simulink model "Clase_parcial_2_control_2"  (R2016a)
settings: Solver=VariableStepAuto  StartTime=0.0  StopTime=10.0  RelTol=1e-3
values from neighbouring files (symbols this model uses):
  A = [0,1;19,1]    [Control_sist_no_lineal_punto_operacion.m]    (also in Datos_Regulador_Segundo_Orden.mat = [-1  0; 0  2]; Metodo_ganancias.m = [0,1;3*x.^2+10*x+6,1]; Metodo_modos_deslizantes.m = [0 1;-12 -7]; Observador_Estados.m = [-1,0;0,2])
  B = [1;2]    [Control_sist_no_lineal_punto_operacion.m]    (also in Datos_Regulador_Segundo_Orden.mat = [1 1]; Metodo_ganancias.m; Metodo_modos_deslizantes.m = [0;1]; Observador_Estados.m = [1;1])
  C = [1,0]    [Control_sist_no_lineal_punto_operacion.m]    (also in Datos_Regulador_Segundo_Orden.mat = [1 1]; Metodo_ganancias.m; Metodo_modos_deslizantes.m = [1 0]; Observador_Estados.m = [1,1])
undefined symbols (not defined in the file or in its folder): k_regulador
settings Model: Creator=Daniel  LastModifiedBy=Daniel

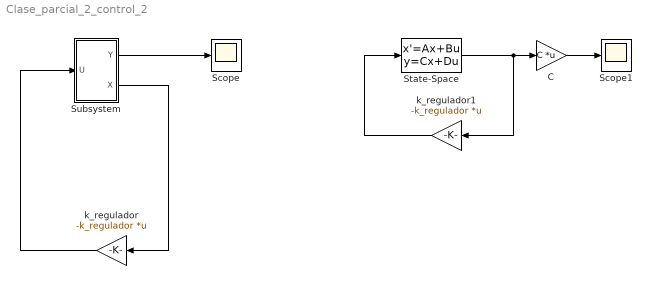
== system Clase_parcial_2_control_2 ==
  C : Gain  Gain=C  Multiplication=Matrix(K*u) (u vector)
  Scope : Scope
  Scope1 : Scope
  State-Space : StateSpace  A=A  B=B  C=eye(2)  D=zeros(2,2)  X0=[1;1]
  Subsystem : Subsystem
  k_regulador : Gain  Gain=-k_regulador  Multiplication=Matrix(K*u) (u vector)
  k_regulador1 : Gain  Gain=-k_regulador  Multiplication=Matrix(K*u) (u vector)
  wires:
  Subsystem/1(Y) -> Scope/1
  k_regulador/1 -> Subsystem/1(U)
  Subsystem/2(X) -> k_regulador/1
  k_regulador1/1 -> State-Space/1
  State-Space/1 -> k_regulador1/1, C/1
  C/1 -> Scope1/1

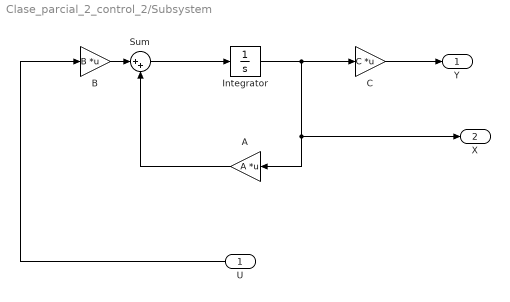
== system Clase_parcial_2_control_2/Subsystem ==
  U : Inport
  A : Gain  Gain=A  Multiplication=Matrix(K*u) (u vector)
  B : Gain  Gain=B  Multiplication=Matrix(K*u) (u vector)
  C : Gain  Gain=C  Multiplication=Matrix(K*u) (u vector)
  Integrator : Integrator  InitialCondition=[1;1]
  Sum : Sum  Inputs=|++
  Y : Outport
  X : Outport  Port=2
  wires:
  Sum/1 -> Integrator/1
  A/1 -> Sum/2
  U/1 -> B/1
  B/1 -> Sum/1
  C/1 -> Y/1
  Integrator/1 -> X/1, A/1, C/1
